simulink model "Demo_MinSegMotor_RP2040_25a_PI_SpeedControl"  (R2025a)
settings: Solver=FixedStepDiscrete  StartTime=0.0  StopTime=inf  FixedStep=.004  RelTol=1e-3
undefined symbols (not defined in the file): DiscIntNeverNeededParam
libraries: simulink x4, arduinolib x3
settings Model: SILPILModeSetting=veronly  ExtModeTrigDuration=2  Creator=Alec  LastModifiedBy=hurstj
settings SolverCC: AlgebraicLoopSolver=TrustRegion
settings DataIOCC: LimitDataPoints=on  SaveFormat=Array  SaveOutput=off  DSMLogging=off  SaveTime=off  ReturnWorkspaceOutputs=off
settings OptimizationCC: EnhancedBackFolding=on  PassReuseOutputArgsThreshold=0.0  ExpressionDepthLimit=2147483647.0  MaxStackSize=64  OptimizeBlockOrder=speed  DifferentSizesBufferReuse=on  OptimizationCustomize=off
settings DebuggingCC: UnderspecifiedInitializationDetection=Classic  MergeDetectMultiDrivingBlocksExec=none  ParameterTunabilityLossMsg=error  UnconnectedInputMsg=warning  UnconnectedOutputMsg=warning  UnconnectedLineMsg=warning  StateNameClashWarn=warning  SFUnexpectedBacktrackingDiag=warning  SFNoUnconditionalDefaultTransitionDiag=warning  SFExecutionAtInitializationDiag=none  ArithmeticOperatorsInVariantConditions=warning
settings HardwareCC: ProdBitPerPointer=32.0  ProdBitPerSizeT=32.0  ProdBitPerPtrDiffT=32.0  ProdLargestAtomicInteger=Long  ProdLargestAtomicFloat=Double  ProdWordSize=32.0  ProdHWDeviceType=ARM Compatible->ARM Cortex  UseEmbeddedCoderFeatures=off  UseSimulinkCoderFeatures=off
settings ModelReferenceCC: EnableRefExpFcnMdlSchedulingChecks=on  PropagateSignalLabelsOutOfModel=off
settings SFSimCC: SimUseLocalCustomCode=off  MATLABDynamicMemAlloc=off  CustomCodeUndefinedFunction=UseInterfaceOnly
settings RTWCC: SystemTargetFile=ert.tlc  HardwareBoard=Arduino Nano RP2040 Connect  TemplateMakefile=ert_default_tmf  RTWVerbose=off  RTWUseLocalCustomCode=off  Toolchain=Arduino ARM MBED RP2040  BuildConfiguration=Faster Runs  GPUComputeCapability=3.5  DLArmComputeVersion=19.05  Description=Embedded Coder
settings CodeAppCC: ForceParamTrailComments=on  OperatorAnnotations=on  MangleLength=10.0
settings ERTTargetCC: ExtModeTransport=3.0  ExtModeAutomaticAllocSize=off  ExtModeStaticAllocSize=65536.0  InlinedParameterPlacement=Hierarchical  DynamicArrayContainerType=coder::array  ERTCustomFileBanners=off  SupportContinuousTime=on  SupportNonInlinedSFcns=on  RemoveResetFunc=off  SupportVariableSizeSignals=on  ModelStepFunctionPrototypeControlCompliant=off
settings ConfigComp: CovMetricSettings=dw  CovSaveCumulativeToWorkspaceVar=on  CovSaveSingleToWorkspaceVar=on  CovExternalEMLEnable=off

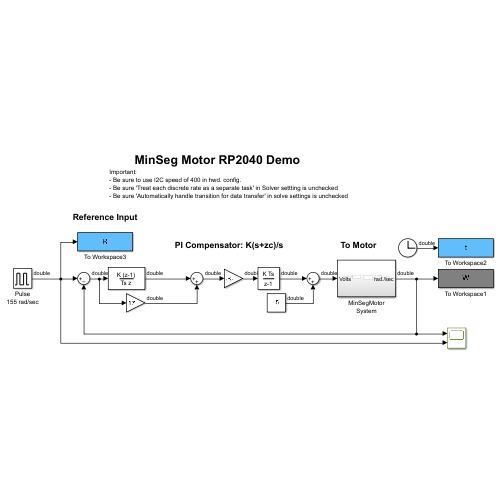
[thumbnail: Simulink's stored preview of the top-level diagram]
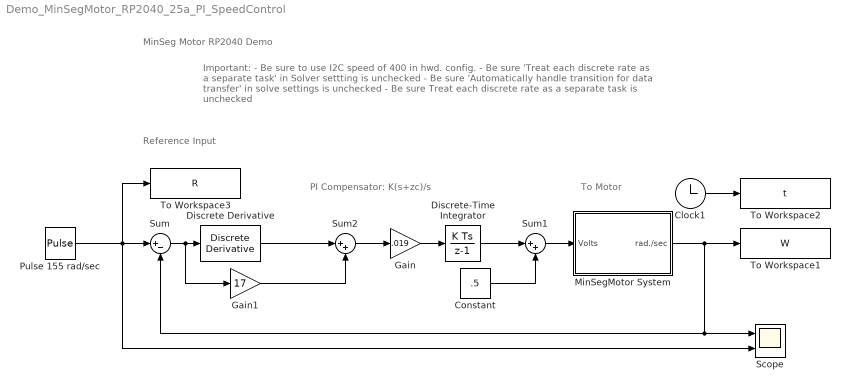
== system Demo_MinSegMotor_RP2040_25a_PI_SpeedControl ==
  note: MinSeg Motor RP2040 Demo
  note: Important:
      | - Be sure to use I2C speed of 400 in hwd. config.
      | - Be sure 'Treat each discrete rate as a separate task' in Solver settting is unchecked
      | - Be sure 'Automatically handle transition for data transfer' in solve settings is unchecked
      | - Be sure Treat each discrete rate as a separate task is unchecked
  note: Reference Input
  note: PI Compensator: K(s+zc)/s
  note: To Motor
  Clock1 : Clock
  Constant : Constant  Value=.5
  Discrete Derivative : simulink/Discrete/Discrete Derivative  gainval=1.0  ICPrevScaledInput=0.0  OutMin=[]  OutMax=[]  OutDataType=fixdt(1, 16)  OutScaling=2^-10  DoSatur=off
  Discrete-Time Integrator : DiscreteIntegrator  SampleTime=-1  ICPrevOutput=DiscIntNeverNeededParam  ICPrevScaledInput=DiscIntNeverNeededParam
  Gain : Gain  Gain=.019
  Gain1 : Gain  Gain=17
  MinSegMotor System : Subsystem
  Pulse 155 rad/sec : DiscretePulseGenerator  PulseType=Time based  Amplitude=155  Period=4  PulseWidth=50
  Scope : Scope  NumInputPorts=2
      settings: ActiveDisplayYMinimum=-21.604328222194336  ActiveDisplayYMaximum=182.68149646388963
  Sum : Sum  Inputs=|+-
  Sum1 : Sum  Inputs=|++
  Sum2 : Sum  Inputs=|++
  To Workspace1 : ToWorkspace  VariableName=W  SampleTime=-1
      settings: Save2DSignal=2-D array (concatenate along first dimension)
  To Workspace2 : ToWorkspace  VariableName=t  SampleTime=-1
      settings: Save2DSignal=2-D array (concatenate along first dimension)
  To Workspace3 : ToWorkspace  VariableName=R  SampleTime=-1
      settings: Save2DSignal=2-D array (concatenate along first dimension)
  wires:
  Gain/1 -> Discrete-Time Integrator/1
  Gain1/1 -> Sum2/2
  Constant/1 -> Sum1/2
  Sum/1 -> Gain1/1, Discrete Derivative/1
  Sum1/1 -> MinSegMotor System/1(Volts)
  Discrete Derivative/1 -> Sum2/1
  MinSegMotor System/1(rad./sec) -> To Workspace1/1, Scope/1, Sum/2
  Pulse 155 rad/sec/1 -> Scope/2, To Workspace3/1, Sum/1
  Clock1/1 -> To Workspace2/1
  Discrete-Time Integrator/1 -> Sum1/1
  Sum2/1 -> Gain/1

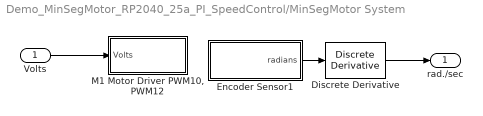
== system Demo_MinSegMotor_RP2040_25a_PI_SpeedControl/MinSegMotor System ==
  Volts : Inport
  Discrete Derivative : simulink/Discrete/Discrete Derivative  gainval=1.0  ICPrevScaledInput=0.0  OutMin=[]  OutMax=[]  OutDataType=fixdt(1, 16)  OutScaling=2^-10  DoSatur=off
  Encoder Sensor1 : Subsystem
      mask DialogControl Control2 Prompt: Encoder Counter - unknown units
  "M1 Motor Driver PWM10, PWM12" : Subsystem  mask{Vsupply=4.8, Voffset=0}
      mask prompts: Vsupply "Driver Voltage"
      mask help:
      | Specify driver supply voltage (around 4.9 for USB, 8.7 for 6AA batteries)
      | Specify the Voltage offset (0-Vsupply)
      |
      | Driver supply voltage can be measured direcly by turning the motor fully on (100% duty cycle) and measuring the voltage across the motor leads.  This is the maximum voltage available to the motor and is used to scale from volts to PWM value 0-255.
      |
      | Note this value must be changed if the supply voltage to the driver is changed, for example, by using batteries.
      |
      | Vsupply is the maximum voltage your system is capable of supplying to system given the power supply. It needs to be measured depending on the power supply.
      mask Display:
      | port_label('input',1,'Volts')
      | text(15,5,['Vsupply=' num2str(Vsupply)])
  rad./sec : Outport
  wires:
  Encoder Sensor1/1(radians) -> Discrete Derivative/1
  Volts/1 -> "M1 Motor Driver PWM10, PWM12"/1(Volts)
  Discrete Derivative/1 -> rad./sec/1

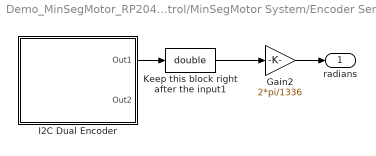
== system Demo_MinSegMotor_RP2040_25a_PI_SpeedControl/MinSegMotor System/Encoder Sensor1 ==
  Gain2 : Gain  Gain=2*pi/1336
  I2C Dual Encoder : Subsystem
  Keep this block right after the input1 : DataTypeConversion  OutDataTypeStr=double  SaturateOnIntegerOverflow=off  RndMeth=Floor
  radians : Outport
  wires:
  Keep this block right after the input1/1 -> Gain2/1
  Gain2/1 -> radians/1
  I2C Dual Encoder/1(Out1) -> Keep this block right after the input1/1

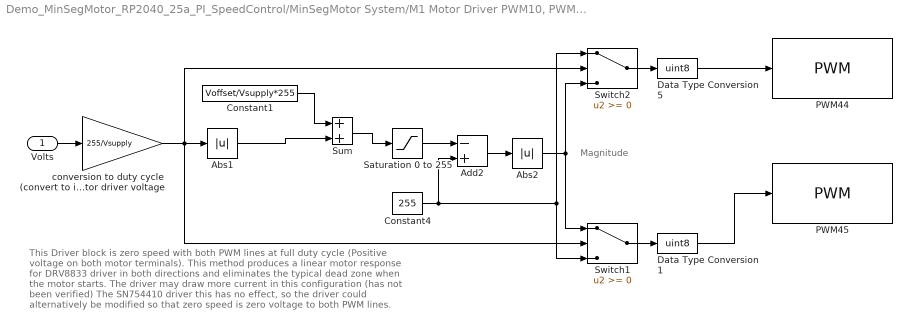
== system Demo_MinSegMotor_RP2040_25a_PI_SpeedControl/MinSegMotor System/M1 Motor Driver PWM10, PWM12 ==
  note: This Driver block is zero speed with both PWM lines at full duty cycle
      |  (Positive voltage on both motor terminals).
      | This method produces a linear motor response for DRV8833 driver
      |  in both directions and eliminates
      | the typical dead zone when the motor starts.
      | The driver may draw more current in this configuration (has not been verified)
      |
      | The SN754410 driver this has no effect, so the driver could alternatively
      | be modified so that zero speed is zero voltage to both PWM lines.
  note: Magnitude
  Volts : Inport
  Abs1 : Abs  SaturateOnIntegerOverflow=off
  Abs2 : Abs  SaturateOnIntegerOverflow=off
  Add2 : Sum  Inputs=-+
  Constant1 : Constant  Value=Voffset/Vsupply*255
  Constant4 : Constant  Value=255
  Data Type Conversion1 : DataTypeConversion  OutDataTypeStr=uint8  SaturateOnIntegerOverflow=off  RndMeth=Floor
  Data Type Conversion5 : DataTypeConversion  OutDataTypeStr=uint8  SaturateOnIntegerOverflow=off  RndMeth=Floor
  PWM44 : arduinolib/PWM  pinNumber=10  frequencyType=Specify  desiredFrequency=4000  achievableFrequency=4000
  PWM45 : arduinolib/PWM  pinNumber=12  frequencyType=Specify  desiredFrequency=4000  achievableFrequency=4000
  Saturation 0 to 255 : Saturate  UpperLimit=255  LowerLimit=0
  Sum : Sum
  Switch1 : Switch  SaturateOnIntegerOverflow=off  InputSameDT=off
  Switch2 : Switch  SaturateOnIntegerOverflow=off  InputSameDT=off
  conversion to duty cycle (convert to int) denominator is motor driver voltage : Gain  Gain=255/Vsupply  OutDataTypeStr=int16
  wires:
  Abs1/1 -> Sum/2
  Sum/1 -> Saturation 0 to 255/1
  Constant1/1 -> Sum/1
  Volts/1 -> conversion to duty cycle (convert to int) denominator is motor driver voltage/1
  conversion to duty cycle (convert to int) denominator is motor driver voltage/1 -> Switch2/2, Abs1/1, Switch1/2
  Saturation 0 to 255/1 -> Add2/1
  Constant4/1 -> Switch1/3, Switch2/1, Add2/2
  Add2/1 -> Abs2/1
  Abs2/1 -> Switch2/3, Switch1/1
  Switch2/1 -> Data Type Conversion5/1
  Switch1/1 -> Data Type Conversion1/1
  Data Type Conversion5/1 -> PWM44/1
  Data Type Conversion1/1 -> PWM45/1

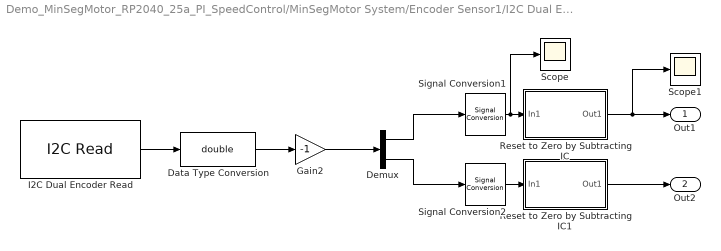
== system Demo_MinSegMotor_RP2040_25a_PI_SpeedControl/MinSegMotor System/Encoder Sensor1/I2C Dual Encoder ==
  Data Type Conversion : DataTypeConversion  OutDataTypeStr=double  SaturateOnIntegerOverflow=off  RndMeth=Floor
  Demux : Demux  Outputs=2
  Gain2 : Gain  Gain=-1
  I2C Dual Encoder Read : arduinolib/I2C Read  I2CModule=0  Mode=Master  SlaveAddress=8  SlaveByteOrder=LittleEndian  Direction=Receiver  RegisterAddressMode=off  RegisterAddress=0  SlaveDataType=int32  DataLength=2  NoAck=off  RepeatedStart=off  OutputStatus=off  blockPlatform=ARDUINO  SampleTime=-1
  Reset to Zero by Subtracting IC : Subsystem
  Reset to Zero by Subtracting IC1 : Subsystem
  Scope : Scope
      settings: ActiveDisplayYMinimum=-4.5575305E+6  ActiveDisplayYMaximum=-4.4059855E+6
  Scope1 : Scope
      settings: ActiveDisplayYMinimum=-15154.375  ActiveDisplayYMaximum=136389.375  DataLoggingVariableName=ScopeData2
  Signal Conversion1 : SignalConversion  OverrideOpt=off
  Signal Conversion2 : SignalConversion  OverrideOpt=off
  Out1 : Outport
  Out2 : Outport  Port=2
  wires:
  Demux/2 -> Signal Conversion2/1
  Signal Conversion1/1 -> Scope/1, Reset to Zero by Subtracting IC/1(In1)
  Signal Conversion2/1 -> Reset to Zero by Subtracting IC1/1(In1)
  Gain2/1 -> Demux/1
  Demux/1 -> Signal Conversion1/1
  I2C Dual Encoder Read/1 -> Data Type Conversion/1
  Data Type Conversion/1 -> Gain2/1
  Reset to Zero by Subtracting IC/1(Out1) -> Scope1/1, Out1/1
  Reset to Zero by Subtracting IC1/1(Out1) -> Out2/1

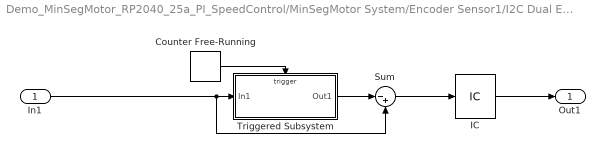
== system Demo_MinSegMotor_RP2040_25a_PI_SpeedControl/MinSegMotor System/Encoder Sensor1/I2C Dual Encoder/Reset to Zero by Subtracting IC ==
  In1 : Inport
  Counter Free-Running : simulink/Sources/Counter Free-Running  NumBits=32  tsamp=-1
  IC : InitialCondition  Value=0
  Sum : Sum  Inputs=|-+
  Triggered Subsystem : Subsystem  TreatAsAtomicUnit=on
  Out1 : Outport
  wires:
  Counter Free-Running/1 -> Triggered Subsystem/Trigger
  Triggered Subsystem/1(Out1) -> Sum/1
  In1/1 -> Sum/2, Triggered Subsystem/1(In1)
  Sum/1 -> IC/1
  IC/1 -> Out1/1

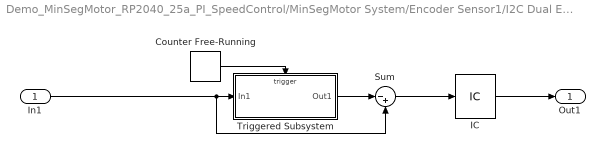
== system Demo_MinSegMotor_RP2040_25a_PI_SpeedControl/MinSegMotor System/Encoder Sensor1/I2C Dual Encoder/Reset to Zero by Subtracting IC1 ==
  In1 : Inport
  Counter Free-Running : simulink/Sources/Counter Free-Running  NumBits=32  tsamp=-1
  IC : InitialCondition  Value=0
  Sum : Sum  Inputs=|-+
  Triggered Subsystem : Subsystem  TreatAsAtomicUnit=on
  Out1 : Outport
  wires:
  Counter Free-Running/1 -> Triggered Subsystem/Trigger
  Triggered Subsystem/1(Out1) -> Sum/1
  In1/1 -> Sum/2, Triggered Subsystem/1(In1)
  Sum/1 -> IC/1
  IC/1 -> Out1/1

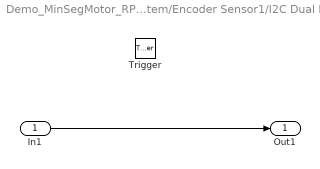
== system Demo_MinSegMotor_RP2040_25a_PI_SpeedControl/MinSegMotor System/Encoder Sensor1/I2C Dual Encoder/Reset to Zero by Subtracting IC/Triggered Subsystem ==
  In1 : Inport
  Trigger : TriggerPort  VariantControl=(inherit)
  Out1 : Outport
  wires:
  In1/1 -> Out1/1

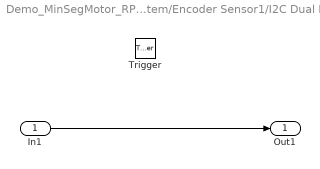
== system Demo_MinSegMotor_RP2040_25a_PI_SpeedControl/MinSegMotor System/Encoder Sensor1/I2C Dual Encoder/Reset to Zero by Subtracting IC1/Triggered Subsystem ==
  In1 : Inport
  Trigger : TriggerPort  VariantControl=(inherit)
  Out1 : Outport
  wires:
  In1/1 -> Out1/1
